simulink model "Offline_TriAxialModulusExtractor"  (R2019a)
settings: Solver=FixedStepDiscrete  StartTime=0.0  StopTime=param_sim_time  FixedStep=1/fs  MaxStep=1/fs  RelTol=1e-3
undefined symbols (not defined in the file): fs
settings Model: PacingRate=100  Creator=rcord  LastModifiedBy=rcord
settings SolverCC: ZeroCrossControl=DisableAll
settings DataIOCC: ExternalInput=[t, scg.input_xyz]  LoadExternalInput=on  SignalLogging=off  DSMLogging=off  SaveTime=off  ReturnWorkspaceOutputs=off  TimeSaveName=t_preprocessing  OutputSaveName=out_preprocessing  LoggingIntervals=[-inf,inf]

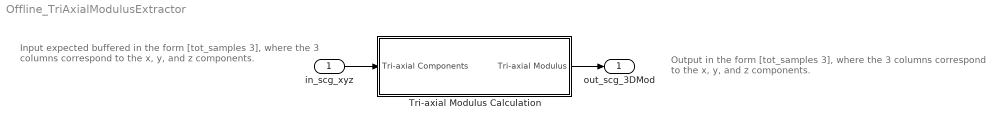
== system Offline_TriAxialModulusExtractor ==
  note: Input expected buffered in the form [tot_samples 3],
      | where the 3 columns correspond to the x, y, and z components.
  note: Output in the form [tot_samples 3],
      | where the 3 columns correspond to the x, y, and z components.
  in_scg_xyz : Inport  SampleTime=1/fs
  Tri-axial Modulus Calculation : Subsystem
  out_scg_3DMod : Outport
  wires:
  Tri-axial Modulus Calculation/1(Tri-axial Modulus) -> out_scg_3DMod/1
  in_scg_xyz/1 -> Tri-axial Modulus Calculation/1(Tri-axial Components)

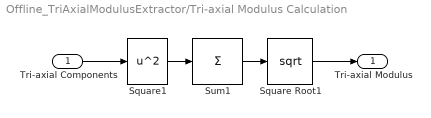
== system Offline_TriAxialModulusExtractor/Tri-axial Modulus Calculation ==
  Tri-axial Components : Inport
  Square Root1 : Sqrt  SaturateOnIntegerOverflow=on
  Square1 : Math  Operator=square  SaturateOnIntegerOverflow=on
  Sum1 : Sum  Inputs=+  CollapseMode=Specified dimension  CollapseDim=2
  Tri-axial Modulus : Outport
  wires:
  Square1/1 -> Sum1/1
  Sum1/1 -> Square Root1/1
  Tri-axial Components/1 -> Square1/1
  Square Root1/1 -> Tri-axial Modulus/1
